simulink model "Tarea_Ejercicio9c_03_04_17"  (R2013a)
settings: Solver=ode45  SolverMode=SingleTasking  StartTime=0.0  StopTime=10.0  RelTol=1e-3
libraries: powerlib x15, powerlib_meascontrol x5
settings Model: Creator=Juan José  LastModifiedBy=Miguel
settings DataIOCC: SignalLoggingSaveFormat=ModelDataLogs
settings OptimizationCC: BlockReduction=off  BooleanDataType=off
settings DebuggingCC: SaveWithParameterizedLinksMsg=none  SignalResolutionControl=TryResolveAllWithWarning  SolverPrmCheckMsg=none  MultiTaskDSMMsg=warning  MultiTaskCondExecSysMsg=none  StrictBusMsg=None
settings HardwareCC: TargetUnknown=on
settings RTWCC: IncludeERTFirstTime=on

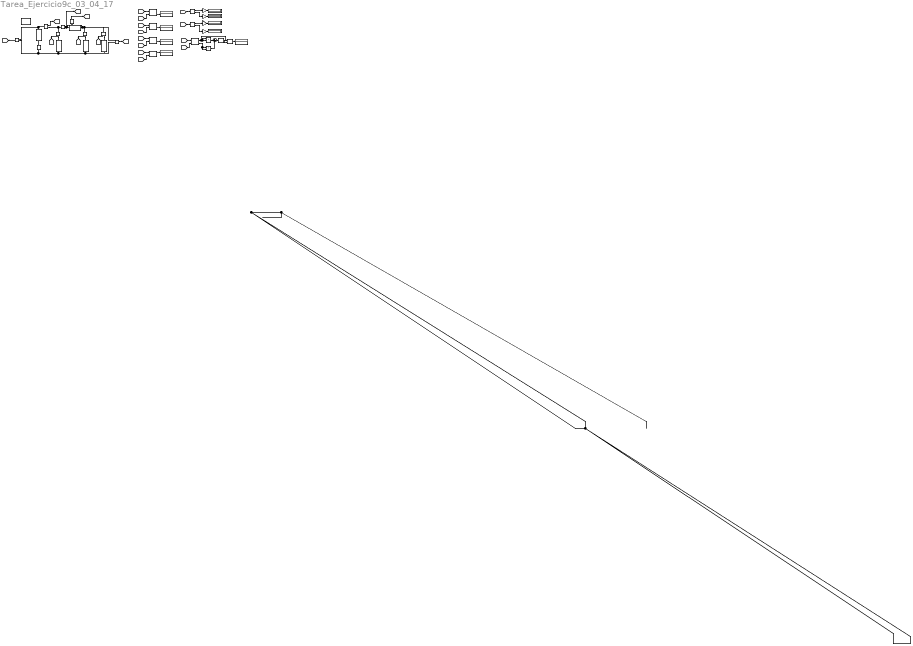
== system Tarea_Ejercicio9c_03_04_17 ==
  AC Voltage Source1 : powerlib/Electrical Sources/AC Voltage Source  Amplitude=200*sqrt(2)  Phase=0  Frequency=50  SampleTime=0  Measurements=None
  Complex to Magnitude-Angle2 : ComplexToMagnitudeAngle
  Complex to Magnitude-Angle3 : ComplexToMagnitudeAngle
  Current Measurement{,1..2,4..5} (5 alike) : powerlib/Measurements/Current Measurement  PhasorSimulation=on  OutputType=Complex  PSBequivalent=0
  Display{1..2,4,6..7,9..12} (9 alike) : Display
      Display10 settings: Decimation=6
      Display9 settings: Decimation=6
  Divide : Product  Inputs=*/
  Gain2 : Gain  Gain=180/pi
  Gain3 : Gain  Gain=180/pi
  Gain4 : Gain  Gain=1/sqrt(2)
  Gain5 : Gain  Gain=1/sqrt(2)
  Power (Phasor){1..2,4..6} (5 alike) : powerlib_meascontrol/Measurements/Power (Phasor)
  Product : Product
  Product1 : Product
  Series RLC Branch : powerlib/Elements/Series RLC Branch  LConnTagsString=__new0  RConnTagsString=__new0  BranchType=R  Resistance=41.3793  Inductance=3/(2*pi*60)  SetiL0=off  InitialCurrent=0  Capacitance=1e-6  Setx0=off  InitialVoltage=0  Measurements=None
  Series RLC Branch1 : powerlib/Elements/Series RLC Branch  LConnTagsString=__new0  RConnTagsString=__new0  BranchType=R  Resistance=1e-3  Inductance=3/(2*pi*60)  SetiL0=off  InitialCurrent=0  Capacitance=1e-6  Setx0=off  InitialVoltage=0  Measurements=None
  Series RLC Branch2 : powerlib/Elements/Series RLC Branch  LConnTagsString=__new0  RConnTagsString=__new0  BranchType=C  Resistance=4  Inductance=3/(2*pi*60)  SetiL0=off  InitialCurrent=0  Capacitance=4.414189153e-5  Setx0=off  InitialVoltage=0  Measurements=None
  Series RLC Branch3 : powerlib/Elements/Series RLC Branch  LConnTagsString=__new0  RConnTagsString=__new0  BranchType=L  Resistance=4  Inductance=0.219524  SetiL0=off  InitialCurrent=0  Capacitance=1e-6  Setx0=off  InitialVoltage=0  Measurements=None
  Series RLC Branch5 : powerlib/Elements/Series RLC Branch  LConnTagsString=__new0  RConnTagsString=__new0  BranchType=C  Resistance=4  Inductance=3/(2*pi*60)  SetiL0=off  InitialCurrent=0  Capacitance=7.692486e-5  Setx0=off  InitialVoltage=0  Measurements=None
  Sqrt : Sqrt  SaturateOnIntegerOverflow=on
  Sum : Sum  Inputs=|++
  Voltage Measurement1 : powerlib/Measurements/Voltage Measurement  PhasorSimulation=on  OutputType=Complex  PSBequivalent=0
  Voltage Measurement2 : powerlib/Measurements/Voltage Measurement  PhasorSimulation=on  OutputType=Complex  PSBequivalent=0
  Voltage Measurement4 : powerlib/Measurements/Voltage Measurement  PhasorSimulation=on  OutputType=Complex  PSBequivalent=0
  powergui : powerlib/powergui  Priority=1  SimulationMode=Phasor  SolverType=Tustin  SampleTime=50e-6  frequency=50  SPID=off  DisableSnubberDevices=off  DisableRonSwitches=off  DisableVfSwitches=off  SwTol=0  Interpol=off  DisplayEquations=off  frequencyindice=50  Pbase=100e6  ErrMax=1e-4  Iterations=50  UnitsV=kV  UnitsW=MW  FunctionMessages=off  echomessages=off  HookPort=off  EnableUseOfTLC=off  x0status=blocks  RestoreLinks=warning  ResistiveCurrentMeasurement=off  Frange=[0:2:500]  Ylog=off  Xlog=on  ShowGrid=off  save=off  variable=ZData  structure=0  ZoomFFT=off  StartTime=0.0  cycles=1  DisplayStyle=1  fundamental=60  FreqAxis=off  MaxFrequency=1000  frequencyindicesteady=1  RmsSteady=1  display=off  Ts=100  methode=off
  wires:
  Current Measurement1/1 -> [IC1]
  Current Measurement4/1 -> [IC2]
  Current Measurement5/1 -> [IR]
  Current Measurement/1 -> [IL]
  Voltage Measurement2/1 -> [VL]
  Voltage Measurement1/1 -> [V]
  Voltage Measurement4/1 -> [VC2]
  [V] -> Power (Phasor)1/1
  [IC1] -> Power (Phasor)1/2
  Power (Phasor)1/2 -> Display1/1
  [VL] -> Power (Phasor)2/1
  [IL] -> Power (Phasor)2/2
  Power (Phasor)2/2 -> Display4/1
  [VC2] -> Power (Phasor)4/1
  [IC2] -> Power (Phasor)4/2
  Power (Phasor)4/2 -> Display6/1
  Power (Phasor)5/1 -> Display7/1
  [VC2] -> Power (Phasor)5/1
  [IR] -> Power (Phasor)5/2
  Complex to Magnitude-Angle2/2 -> Gain3/1
  [VC2] -> Complex to Magnitude-Angle3/1
  Complex to Magnitude-Angle3/1 -> Gain5/1
  Complex to Magnitude-Angle3/2 -> Gain2/1
  Gain2/1 -> Display11/1
  Gain3/1 -> Display10/1
  [IL] -> Complex to Magnitude-Angle2/1
  Complex to Magnitude-Angle2/1 -> Gain4/1
  Gain5/1 -> Display12/1
  Gain4/1 -> Display9/1
  [V] -> Power (Phasor)6/1
  [I] -> Power (Phasor)6/2
  Current Measurement2/1 -> [I]
  Power (Phasor)6/1 -> Divide/1, Product/1, Product/2
  Power (Phasor)6/2 -> Product1/2, Product1/1
  Product/1 -> Sum/1
  Product1/1 -> Sum/2
  Sum/1 -> Sqrt/1
  Sqrt/1 -> Divide/2
  Divide/1 -> Display2/1
  connections:
  AC Voltage Source1/RConn1 -- Series RLC Branch1/RConn1
  Voltage Measurement1/LConn1 -- Current Measurement2/LConn1 -- Series RLC Branch1/LConn1
  Current Measurement/RConn1 -- Voltage Measurement2/LConn1 -- Series RLC Branch3/LConn1
  Series RLC Branch2/RConn1 -- Series RLC Branch/RConn1 -- Voltage Measurement4/LConn2 -- Series RLC Branch5/RConn1 -- Voltage Measurement1/LConn2 -- AC Voltage Source1/LConn1
  Current Measurement1/RConn1 -- Series RLC Branch2/LConn1
  Current Measurement4/RConn1 -- Series RLC Branch5/LConn1
  Current Measurement5/RConn1 -- Series RLC Branch/LConn1
  Current Measurement4/LConn1 -- Voltage Measurement4/LConn1 -- Current Measurement5/LConn1 -- Voltage Measurement2/LConn2 -- Series RLC Branch3/RConn1
  ?
  Current Measurement1/LConn1 -- Current Measurement2/RConn1 -- Current Measurement/LConn1
